simulink model "coefficients"  (R2022b)
settings: Solver=VariableStepAuto  StartTime=0.0  StopTime=10.0  RelTol=1e-3
undefined symbols (not defined in the file): simdb
settings Model: Creator=David  LastModifiedBy=David

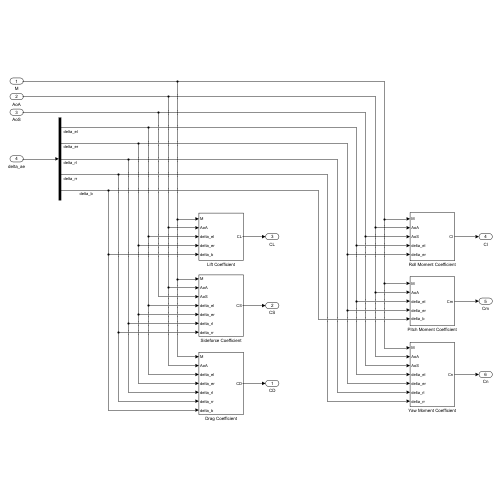
[thumbnail: Simulink's stored preview of the top-level diagram]
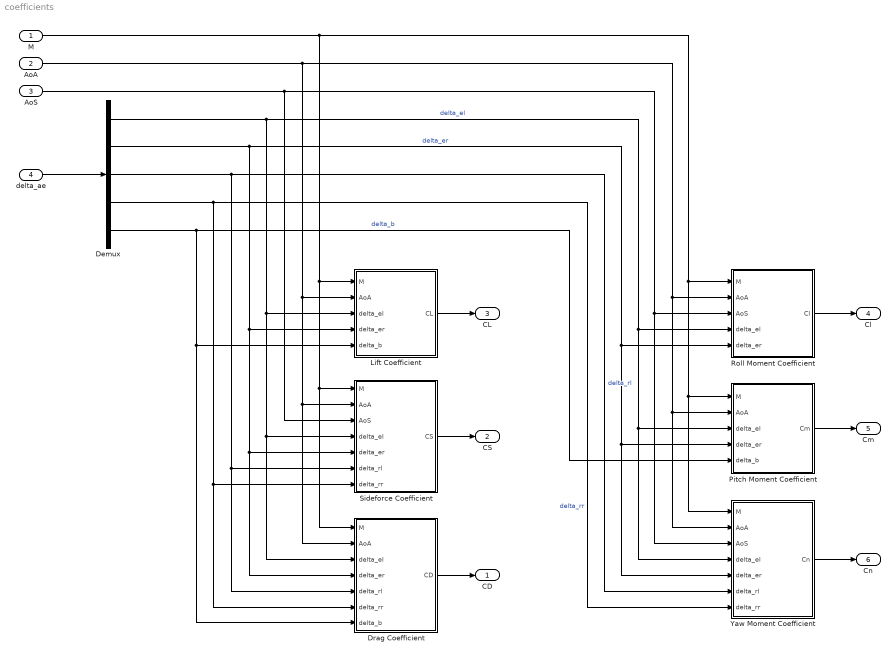
== system coefficients ==
  M : Inport
  AoA : Inport  Port=2
  AoS : Inport  Port=3
  delta_ae : Inport  Port=4
  Demux : Demux  Outputs=5
  Drag Coefficient : Subsystem
  Lift Coefficient : Subsystem
  Pitch Moment Coefficient : Subsystem
  Roll Moment Coefficient : Subsystem
  Sideforce Coefficient : Subsystem
  Yaw Moment Coefficient : Subsystem
  CD : Outport
  CS : Outport  Port=2
  CL : Outport  Port=3
  Cl : Outport  Port=4
  Cm : Outport  Port=5
  Cn : Outport  Port=6
  wires:
  delta_ae/1 -> Demux/1
  Demux/1 -> Drag Coefficient/3(delta_el), Sideforce Coefficient/4(delta_el), Lift Coefficient/3(delta_el), Yaw Moment Coefficient/4(delta_el), Pitch Moment Coefficient/3(delta_el), Roll Moment Coefficient/4(delta_el)  "delta_el"
  Demux/2 -> Pitch Moment Coefficient/4(delta_er), Yaw Moment Coefficient/5(delta_er), Roll Moment Coefficient/5(delta_er), Drag Coefficient/4(delta_er), Sideforce Coefficient/5(delta_er), Lift Coefficient/4(delta_er)  "delta_er"
  Demux/5 -> Drag Coefficient/7(delta_b), Lift Coefficient/5(delta_b), Pitch Moment Coefficient/5(delta_b)  "delta_b"
  M/1 -> Yaw Moment Coefficient/1(M), Pitch Moment Coefficient/1(M), Roll Moment Coefficient/1(M), Drag Coefficient/1(M), Sideforce Coefficient/1(M), Lift Coefficient/1(M)
  AoA/1 -> Drag Coefficient/2(AoA), Sideforce Coefficient/2(AoA), Lift Coefficient/2(AoA), Yaw Moment Coefficient/2(AoA), Pitch Moment Coefficient/2(AoA), Roll Moment Coefficient/2(AoA)
  Demux/3 -> Sideforce Coefficient/6(delta_rl), Drag Coefficient/5(delta_rl), Yaw Moment Coefficient/6(delta_rl)  "delta_rl"
  Demux/4 -> Yaw Moment Coefficient/7(delta_rr), Drag Coefficient/6(delta_rr), Sideforce Coefficient/7(delta_rr)  "delta_rr"
  AoS/1 -> Sideforce Coefficient/3(AoS), Yaw Moment Coefficient/3(AoS), Roll Moment Coefficient/3(AoS)
  Lift Coefficient/1(CL) -> CL/1
  Sideforce Coefficient/1(CS) -> CS/1
  Drag Coefficient/1(CD) -> CD/1
  Roll Moment Coefficient/1(Cl) -> Cl/1
  Pitch Moment Coefficient/1(Cm) -> Cm/1
  Yaw Moment Coefficient/1(Cn) -> Cn/1

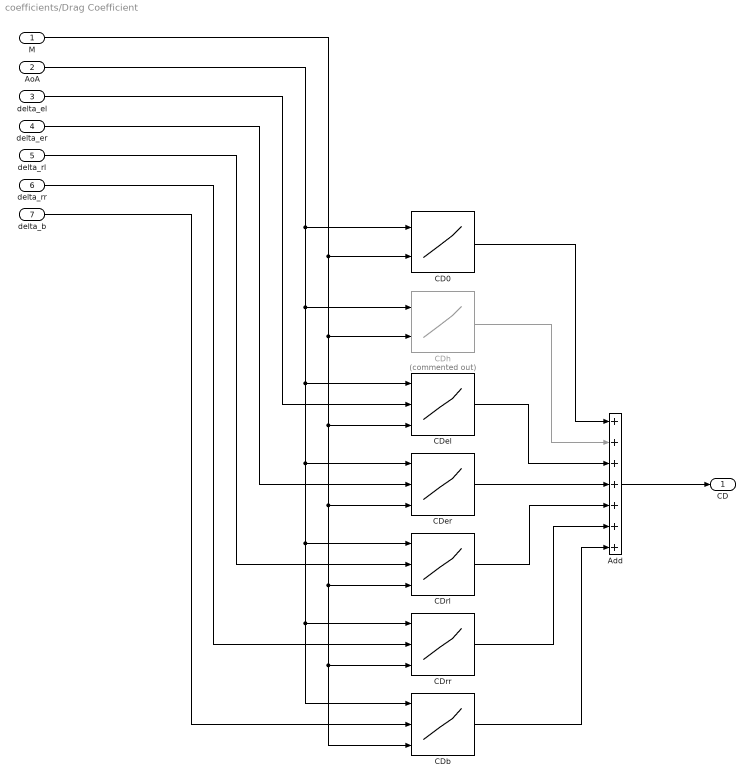
== system coefficients/Drag Coefficient ==
  M : Inport
  AoA : Inport  Port=2
  delta_el : Inport  Port=3
  delta_er : Inport  Port=4
  delta_rl : Inport  Port=5
  delta_rr : Inport  Port=6
  delta_b : Inport  Port=7
  Add : Sum  Inputs=+++++++
  CD0 : Lookup_n-D  BreakpointsForDimension1=simdb.aero.AoA_table  BreakpointsForDimension2=simdb.aero.M_table  Table=simdb.aero.CD0  InterpMethod=Cubic spline  InternalRulePriority=Speed  RndMeth=Simplest
      settings: InputPortMap=u0,u1
  CDb : Lookup_n-D  NumberOfTableDimensions=3  BreakpointsForDimension1=simdb.aero.AoA_table  BreakpointsForDimension2=simdb.aero.delta_b_table  BreakpointsForDimension3=simdb.aero.M_table  Table=simdb.aero.CDb  InterpMethod=Cubic spline  InternalRulePriority=Speed  RndMeth=Simplest
      settings: InputPortMap=u0,u1,u2
  CDel : Lookup_n-D  NumberOfTableDimensions=3  BreakpointsForDimension1=simdb.aero.AoA_table  BreakpointsForDimension2=simdb.aero.delta_el_table  BreakpointsForDimension3=simdb.aero.M_table  Table=simdb.aero.CDel  InterpMethod=Cubic spline  InternalRulePriority=Speed  RndMeth=Simplest
      settings: InputPortMap=u0,u1,u2
  CDer : Lookup_n-D  NumberOfTableDimensions=3  BreakpointsForDimension1=simdb.aero.AoA_table  BreakpointsForDimension2=simdb.aero.delta_el_table  BreakpointsForDimension3=simdb.aero.M_table  Table=simdb.aero.CDel  InterpMethod=Cubic spline  InternalRulePriority=Speed  RndMeth=Simplest
      settings: InputPortMap=u0,u1,u2
  CDh : Lookup_n-D  Commented=on  BreakpointsForDimension1=simdb.aero.AoA_table  BreakpointsForDimension2=simdb.aero.M_table  Table=simdb.aero.CDh  InterpMethod=Cubic spline  InternalRulePriority=Speed  RndMeth=Simplest
      settings: InputPortMap=u0,u1
  CDrl : Lookup_n-D  NumberOfTableDimensions=3  BreakpointsForDimension1=simdb.aero.AoA_table  BreakpointsForDimension2=simdb.aero.delta_rl_table  BreakpointsForDimension3=simdb.aero.M_table  Table=simdb.aero.CDrl  InterpMethod=Cubic spline  InternalRulePriority=Speed  RndMeth=Simplest
      settings: InputPortMap=u0,u1,u2
  CDrr : Lookup_n-D  NumberOfTableDimensions=3  BreakpointsForDimension1=simdb.aero.AoA_table  BreakpointsForDimension2=simdb.aero.delta_rl_table  BreakpointsForDimension3=simdb.aero.M_table  Table=simdb.aero.CDrl  InterpMethod=Cubic spline  InternalRulePriority=Speed  RndMeth=Simplest
      settings: InputPortMap=u0,u1,u2
  CD : Outport
  wires:
  M/1 -> CDrl/3, CDrr/3, CDb/3, CDer/3, CDel/3, CDh/2, CD0/2
  AoA/1 -> CDh/1, CDel/1, CDb/1, CDrr/1, CDrl/1, CDer/1, CD0/1
  delta_el/1 -> CDel/2
  delta_er/1 -> CDer/2
  delta_rl/1 -> CDrl/2
  delta_rr/1 -> CDrr/2
  delta_b/1 -> CDb/2
  CDer/1 -> Add/4
  CDel/1 -> Add/3
  CDh/1 -> Add/2
  CD0/1 -> Add/1
  CDrl/1 -> Add/5
  CDrr/1 -> Add/6
  CDb/1 -> Add/7
  Add/1 -> CD/1

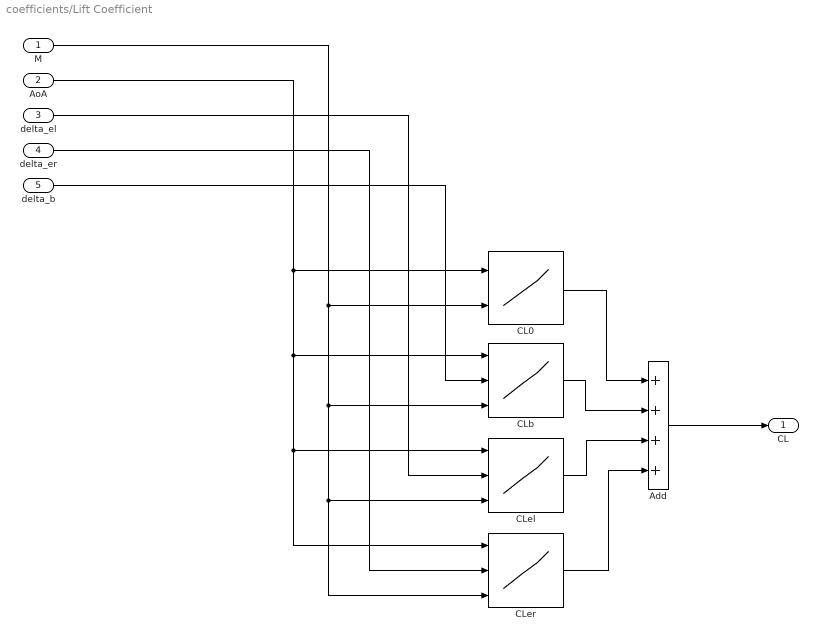
== system coefficients/Lift Coefficient ==
  M : Inport
  AoA : Inport  Port=2
  delta_el : Inport  Port=3
  delta_er : Inport  Port=4
  delta_b : Inport  Port=5
  Add : Sum  Inputs=++++
  CL0 : Lookup_n-D  BreakpointsForDimension1=simdb.aero.AoA_table  BreakpointsForDimension2=simdb.aero.M_table  Table=simdb.aero.CL0  InterpMethod=Cubic spline  InternalRulePriority=Speed  RndMeth=Simplest
      settings: InputPortMap=u0,u1
  CLb : Lookup_n-D  NumberOfTableDimensions=3  BreakpointsForDimension1=simdb.aero.AoA_table  BreakpointsForDimension2=simdb.aero.delta_b_table  BreakpointsForDimension3=simdb.aero.M_table  Table=simdb.aero.CLb  InterpMethod=Cubic spline  InternalRulePriority=Speed  RndMeth=Simplest
      settings: InputPortMap=u0,u1,u2
  CLel : Lookup_n-D  NumberOfTableDimensions=3  BreakpointsForDimension1=simdb.aero.AoA_table  BreakpointsForDimension2=simdb.aero.delta_el_table  BreakpointsForDimension3=simdb.aero.M_table  Table=simdb.aero.CLel  InterpMethod=Cubic spline  InternalRulePriority=Speed  RndMeth=Simplest
      settings: InputPortMap=u0,u1,u2
  CLer : Lookup_n-D  NumberOfTableDimensions=3  BreakpointsForDimension1=simdb.aero.AoA_table  BreakpointsForDimension2=simdb.aero.delta_el_table  BreakpointsForDimension3=simdb.aero.M_table  Table=simdb.aero.CLel  InterpMethod=Cubic spline  InternalRulePriority=Speed  RndMeth=Simplest
      settings: InputPortMap=u0,u1,u2
  CL : Outport
  wires:
  CL0/1 -> Add/1
  M/1 -> CLer/3, CLel/3, CLb/3, CL0/2
  CLb/1 -> Add/2
  AoA/1 -> CL0/1, CLer/1, CLel/1, CLb/1
  CLel/1 -> Add/3
  CLer/1 -> Add/4
  Add/1 -> CL/1
  delta_b/1 -> CLb/2
  delta_er/1 -> CLer/2
  delta_el/1 -> CLel/2

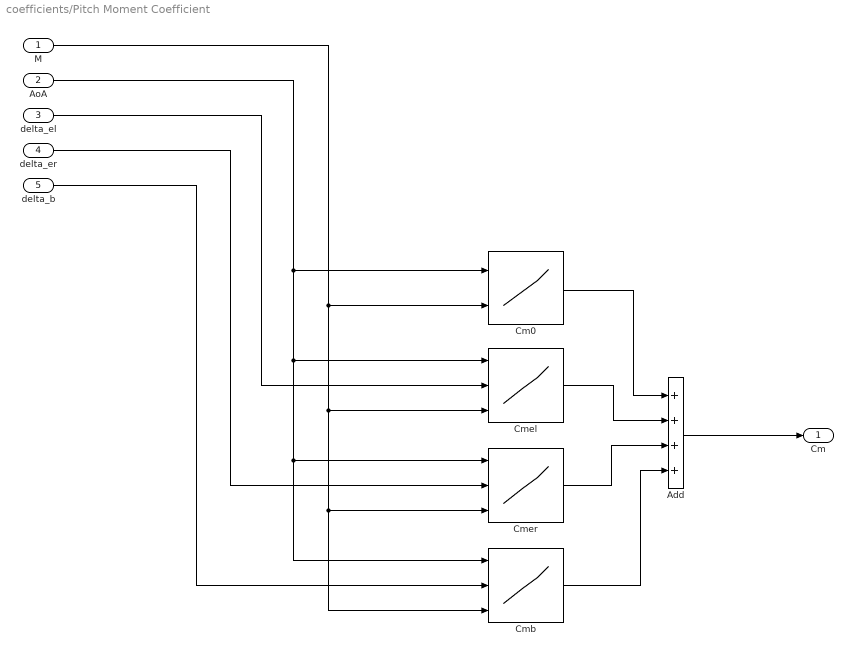
== system coefficients/Pitch Moment Coefficient ==
  M : Inport
  AoA : Inport  Port=2
  delta_el : Inport  Port=3
  delta_er : Inport  Port=4
  delta_b : Inport  Port=5
  Add : Sum  Inputs=++++
  Cm0 : Lookup_n-D  BreakpointsForDimension1=simdb.aero.AoA_table  BreakpointsForDimension2=simdb.aero.M_table  Table=simdb.aero.Clb0  InterpMethod=Cubic spline  InternalRulePriority=Speed  RndMeth=Simplest
      settings: InputPortMap=u0,u1
  Cmb : Lookup_n-D  NumberOfTableDimensions=3  BreakpointsForDimension1=simdb.aero.AoA_table  BreakpointsForDimension2=simdb.aero.delta_b_table  BreakpointsForDimension3=simdb.aero.M_table  Table=simdb.aero.Cmb  InterpMethod=Cubic spline  InternalRulePriority=Speed  RndMeth=Simplest
      settings: InputPortMap=u0,u1,u2
  Cmel : Lookup_n-D  NumberOfTableDimensions=3  BreakpointsForDimension1=simdb.aero.AoA_table  BreakpointsForDimension2=simdb.aero.delta_el_table  BreakpointsForDimension3=simdb.aero.M_table  Table=simdb.aero.Cmel  InterpMethod=Cubic spline  InternalRulePriority=Speed  RndMeth=Simplest
      settings: InputPortMap=u0,u1,u2
  Cmer : Lookup_n-D  NumberOfTableDimensions=3  BreakpointsForDimension1=simdb.aero.AoA_table  BreakpointsForDimension2=simdb.aero.delta_el_table  BreakpointsForDimension3=simdb.aero.M_table  Table=simdb.aero.Cmel  InterpMethod=Cubic spline  InternalRulePriority=Speed  RndMeth=Simplest
      settings: InputPortMap=u0,u1,u2
  Cm : Outport
  wires:
  M/1 -> Cmer/3, Cmb/3, Cmel/3, Cm0/2
  AoA/1 -> Cmb/1, Cmer/1, Cmel/1, Cm0/1
  delta_el/1 -> Cmel/2
  delta_er/1 -> Cmer/2
  delta_b/1 -> Cmb/2
  Add/1 -> Cm/1
  Cm0/1 -> Add/1
  Cmel/1 -> Add/2
  Cmer/1 -> Add/3
  Cmb/1 -> Add/4

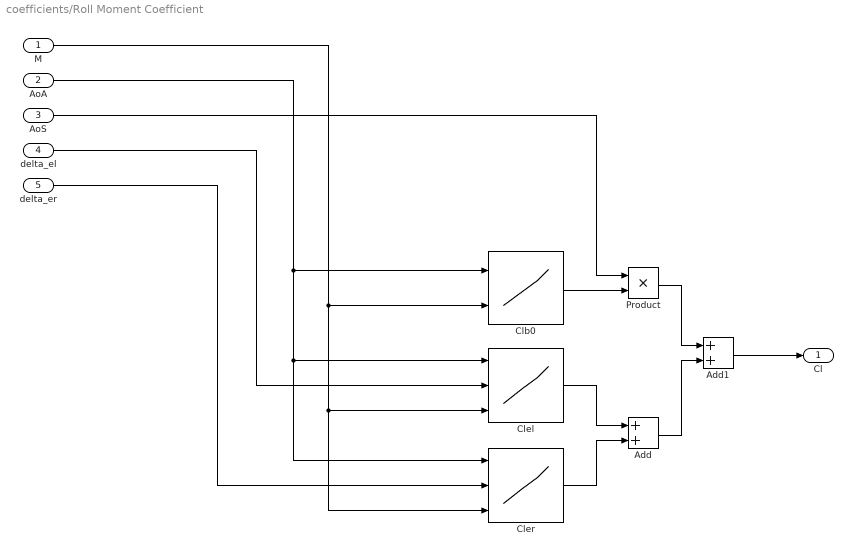
== system coefficients/Roll Moment Coefficient ==
  M : Inport
  AoA : Inport  Port=2
  AoS : Inport  Port=3
  delta_el : Inport  Port=4
  delta_er : Inport  Port=5
  Add : Sum
  Add1 : Sum
  Clb0 : Lookup_n-D  BreakpointsForDimension1=simdb.aero.AoA_table  BreakpointsForDimension2=simdb.aero.M_table  Table=simdb.aero.Clb0  InterpMethod=Cubic spline  InternalRulePriority=Speed  RndMeth=Simplest
      settings: InputPortMap=u0,u1
  Clel : Lookup_n-D  NumberOfTableDimensions=3  BreakpointsForDimension1=simdb.aero.AoA_table  BreakpointsForDimension2=simdb.aero.delta_el_table  BreakpointsForDimension3=simdb.aero.M_table  Table=simdb.aero.Clel  InterpMethod=Cubic spline  InternalRulePriority=Speed  RndMeth=Simplest
      settings: InputPortMap=u0,u1,u2
  Cler : Lookup_n-D  NumberOfTableDimensions=3  BreakpointsForDimension1=simdb.aero.AoA_table  BreakpointsForDimension2=simdb.aero.delta_el_table  BreakpointsForDimension3=simdb.aero.M_table  Table=simdb.aero.Clel  InterpMethod=Cubic spline  InternalRulePriority=Speed  RndMeth=Simplest
      settings: InputPortMap=u0,u1,u2
  Product : Product
  Cl : Outport
  wires:
  M/1 -> Cler/3, Clel/3, Clb0/2
  AoA/1 -> Cler/1, Clel/1, Clb0/1
  delta_el/1 -> Clel/2
  delta_er/1 -> Cler/2
  Clb0/1 -> Product/2
  AoS/1 -> Product/1
  Clel/1 -> Add/1
  Cler/1 -> Add/2
  Add/1 -> Add1/2
  Product/1 -> Add1/1
  Add1/1 -> Cl/1

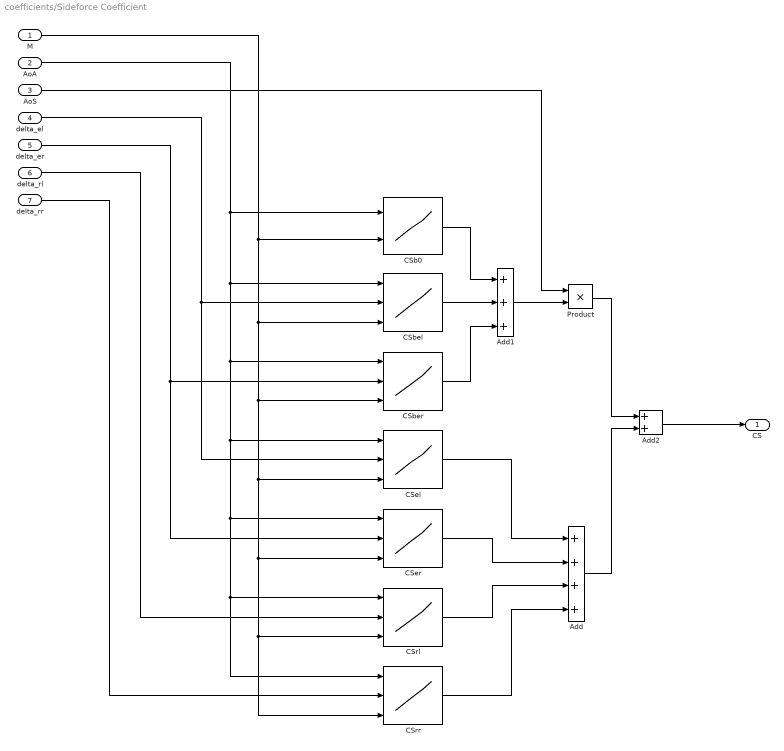
== system coefficients/Sideforce Coefficient ==
  M : Inport
  AoA : Inport  Port=2
  AoS : Inport  Port=3
  delta_el : Inport  Port=4
  delta_er : Inport  Port=5
  delta_rl : Inport  Port=6
  delta_rr : Inport  Port=7
  Add : Sum  Inputs=++++
  Add1 : Sum  Inputs=+++
  Add2 : Sum
  CSb0 : Lookup_n-D  BreakpointsForDimension1=simdb.aero.AoA_table  BreakpointsForDimension2=simdb.aero.M_table  Table=simdb.aero.CSb0  InterpMethod=Cubic spline  InternalRulePriority=Speed  RndMeth=Simplest
      settings: InputPortMap=u0,u1
  CSbel : Lookup_n-D  NumberOfTableDimensions=3  BreakpointsForDimension1=simdb.aero.AoA_table  BreakpointsForDimension2=simdb.aero.delta_el_table  BreakpointsForDimension3=simdb.aero.M_table  Table=simdb.aero.CSbel  InterpMethod=Cubic spline  InternalRulePriority=Speed  RndMeth=Simplest
      settings: InputPortMap=u0,u1,u2
  CSber : Lookup_n-D  NumberOfTableDimensions=3  BreakpointsForDimension1=simdb.aero.AoA_table  BreakpointsForDimension2=simdb.aero.delta_el_table  BreakpointsForDimension3=simdb.aero.M_table  Table=simdb.aero.CSbel  InterpMethod=Cubic spline  InternalRulePriority=Speed  RndMeth=Simplest
      settings: InputPortMap=u0,u1,u2
  CSel : Lookup_n-D  NumberOfTableDimensions=3  BreakpointsForDimension1=simdb.aero.AoA_table  BreakpointsForDimension2=simdb.aero.delta_el_table  BreakpointsForDimension3=simdb.aero.M_table  Table=simdb.aero.CSel  InterpMethod=Cubic spline  InternalRulePriority=Speed  RndMeth=Simplest
      settings: InputPortMap=u0,u1,u2
  CSer : Lookup_n-D  NumberOfTableDimensions=3  BreakpointsForDimension1=simdb.aero.AoA_table  BreakpointsForDimension2=simdb.aero.delta_el_table  BreakpointsForDimension3=simdb.aero.M_table  Table=simdb.aero.CSel  InterpMethod=Cubic spline  InternalRulePriority=Speed  RndMeth=Simplest
      settings: InputPortMap=u0,u1,u2
  CSrl : Lookup_n-D  NumberOfTableDimensions=3  BreakpointsForDimension1=simdb.aero.AoA_table  BreakpointsForDimension2=simdb.aero.delta_rl_table  BreakpointsForDimension3=simdb.aero.M_table  Table=simdb.aero.CSrl  InterpMethod=Cubic spline  InternalRulePriority=Speed  RndMeth=Simplest
      settings: InputPortMap=u0,u1,u2
  CSrr : Lookup_n-D  NumberOfTableDimensions=3  BreakpointsForDimension1=simdb.aero.AoA_table  BreakpointsForDimension2=simdb.aero.delta_rl_table  BreakpointsForDimension3=simdb.aero.M_table  Table=simdb.aero.CSrl  InterpMethod=Cubic spline  InternalRulePriority=Speed  RndMeth=Simplest
      settings: InputPortMap=u0,u1,u2
  Product : Product
  CS : Outport
  wires:
  M/1 -> CSber/3, CSrr/3, CSrl/3, CSer/3, CSel/3, CSbel/3, CSb0/2
  AoA/1 -> CSrr/1, CSrl/1, CSer/1, CSel/1, CSber/1, CSbel/1, CSb0/1
  delta_el/1 -> CSbel/2, CSel/2
  delta_er/1 -> CSer/2, CSber/2
  delta_rl/1 -> CSrl/2
  delta_rr/1 -> CSrr/2
  CSel/1 -> Add/1
  CSer/1 -> Add/2
  CSrl/1 -> Add/3
  CSrr/1 -> Add/4
  CSbel/1 -> Add1/2
  CSber/1 -> Add1/3
  CSb0/1 -> Add1/1
  Add1/1 -> Product/2
  AoS/1 -> Product/1
  Product/1 -> Add2/1
  Add/1 -> Add2/2
  Add2/1 -> CS/1

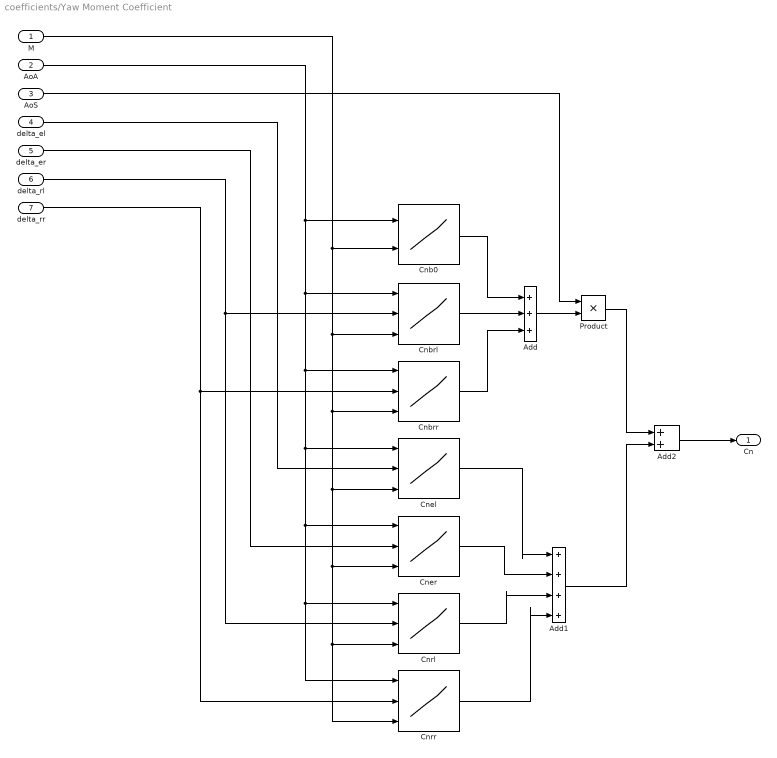
== system coefficients/Yaw Moment Coefficient ==
  M : Inport
  AoA : Inport  Port=2
  AoS : Inport  Port=3
  delta_el : Inport  Port=4
  delta_er : Inport  Port=5
  delta_rl : Inport  Port=6
  delta_rr : Inport  Port=7
  Add : Sum  Inputs=+++
  Add1 : Sum  Inputs=++++
  Add2 : Sum
  Cnb0 : Lookup_n-D  BreakpointsForDimension1=simdb.aero.AoA_table  BreakpointsForDimension2=simdb.aero.M_table  Table=simdb.aero.Clb0  InterpMethod=Cubic spline  InternalRulePriority=Speed  RndMeth=Simplest
      settings: InputPortMap=u0,u1
  Cnbrl : Lookup_n-D  NumberOfTableDimensions=3  BreakpointsForDimension1=simdb.aero.AoA_table  BreakpointsForDimension2=simdb.aero.delta_rl_table  BreakpointsForDimension3=simdb.aero.M_table  Table=simdb.aero.Cnbrl  InterpMethod=Cubic spline  InternalRulePriority=Speed  RndMeth=Simplest
      settings: InputPortMap=u0,u1,u2
  Cnbrr : Lookup_n-D  NumberOfTableDimensions=3  BreakpointsForDimension1=simdb.aero.AoA_table  BreakpointsForDimension2=simdb.aero.delta_rl_table  BreakpointsForDimension3=simdb.aero.M_table  Table=simdb.aero.Cnbrl  InterpMethod=Cubic spline  InternalRulePriority=Speed  RndMeth=Simplest
      settings: InputPortMap=u0,u1,u2
  Cnel : Lookup_n-D  NumberOfTableDimensions=3  BreakpointsForDimension1=simdb.aero.AoA_table  BreakpointsForDimension2=simdb.aero.delta_el_table  BreakpointsForDimension3=simdb.aero.M_table  Table=simdb.aero.Cnel  InterpMethod=Cubic spline  InternalRulePriority=Speed  RndMeth=Simplest
      settings: InputPortMap=u0,u1,u2
  Cner : Lookup_n-D  NumberOfTableDimensions=3  BreakpointsForDimension1=simdb.aero.AoA_table  BreakpointsForDimension2=simdb.aero.delta_el_table  BreakpointsForDimension3=simdb.aero.M_table  Table=simdb.aero.Cnel  InterpMethod=Cubic spline  InternalRulePriority=Speed  RndMeth=Simplest
      settings: InputPortMap=u0,u1,u2
  Cnrl : Lookup_n-D  NumberOfTableDimensions=3  BreakpointsForDimension1=simdb.aero.AoA_table  BreakpointsForDimension2=simdb.aero.delta_rl_table  BreakpointsForDimension3=simdb.aero.M_table  Table=simdb.aero.Cnrl  InterpMethod=Cubic spline  InternalRulePriority=Speed  RndMeth=Simplest
      settings: InputPortMap=u0,u1,u2
  Cnrr : Lookup_n-D  NumberOfTableDimensions=3  BreakpointsForDimension1=simdb.aero.AoA_table  BreakpointsForDimension2=simdb.aero.delta_rl_table  BreakpointsForDimension3=simdb.aero.M_table  Table=simdb.aero.Cnrl  InterpMethod=Cubic spline  InternalRulePriority=Speed  RndMeth=Simplest
      settings: InputPortMap=u0,u1,u2
  Product : Product
  Cn : Outport
  wires:
  M/1 -> Cnb0/2, Cnbrl/3, Cnbrr/3, Cnel/3, Cner/3, Cnrl/3, Cnrr/3
  AoA/1 -> Cnb0/1, Cnbrl/1, Cnbrr/1, Cnel/1, Cner/1, Cnrl/1, Cnrr/1
  delta_el/1 -> Cnel/2
  delta_er/1 -> Cner/2
  delta_rl/1 -> Cnrl/2, Cnbrl/2
  delta_rr/1 -> Cnrr/2, Cnbrr/2
  Cnbrr/1 -> Add/3
  Cnbrl/1 -> Add/2
  Cnb0/1 -> Add/1
  Add/1 -> Product/2
  AoS/1 -> Product/1
  Cnel/1 -> Add1/1
  Cner/1 -> Add1/2
  Cnrl/1 -> Add1/3
  Cnrr/1 -> Add1/4
  Add1/1 -> Add2/2
  Product/1 -> Add2/1
  Add2/1 -> Cn/1
